simulink model "TestSIMapi"  (R2019b)
settings: Solver=ode15s  StartTime=0  StopTime=5  FixedStep=1e-3  RelTol=1e-3
values from neighbouring files (symbols this model uses):
  SimpleOdeModel = nonlinearModel('derivativeFunction',test_func,                       'outputFunction',output_func,                       'theta',[5;1],                       'simTol',1e-7,                       'statSolMethod','sol',                       'nrOfInputs',1,                       'nrOfOutputs',1,                       'nrOfStates',1,                       'freeParamsForOptIdx',[1 2],                  ...(+34 chars)    [SISONonlin.m]    (also in Wheel_Identi.m = nonlinearModel('derivativeFunction',test_func,              )
undefined symbols (not defined in the file or in its folder): x0
settings Model: Creator=ritzberger  LastModifiedBy=ritzberger
settings SolverCC: ZeroCrossAlgorithm=Adaptive
settings DataIOCC: ReturnWorkspaceOutputs=off
settings DebuggingCC: IgnoredZcDiagnostic=none  ArithmeticOperatorsInVariantConditions=warning
settings SFSimCC: SimUseLocalCustomCode=off  CustomCodeUndefinedFunction=UseInterfaceOnly
settings RTWCC: RTWUseLocalCustomCode=off

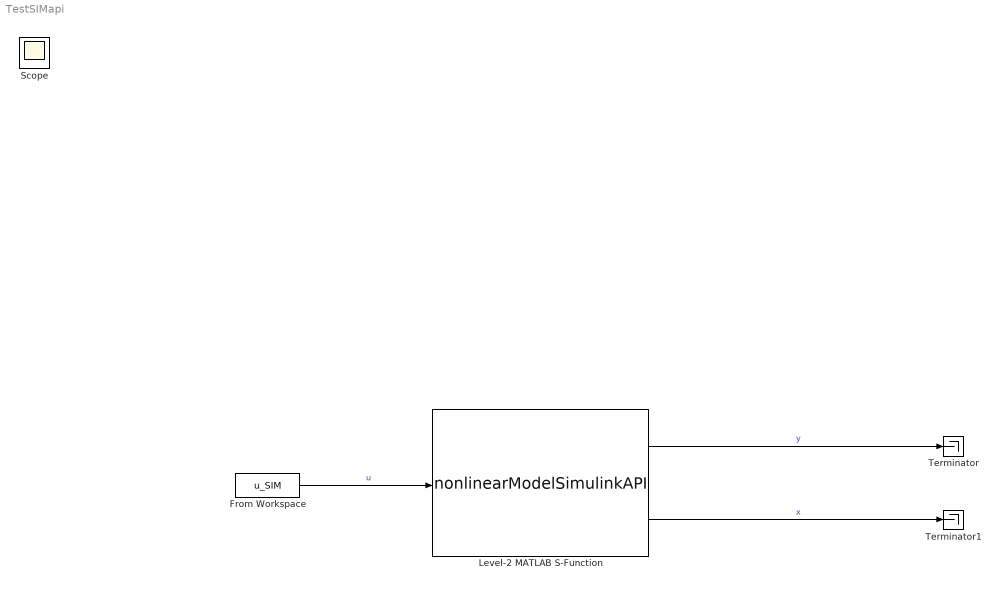
== system TestSIMapi ==
  From Workspace : FromWorkspace  VariableName=u_SIM  SampleTime=0
  Level-2 MATLAB S-Function : M-S-Function  FunctionName=nonlinearModelSimulinkAPI  Parameters=x0,SimpleOdeModel
  Terminator : Terminator
  Terminator1 : Terminator
  Scope : Scope
  wires:
  Level-2 MATLAB S-Function/1 -> Terminator/1  "y"
  Level-2 MATLAB S-Function/2 -> Terminator1/1  "x"
  From Workspace/1 -> Level-2 MATLAB S-Function/1  "u"
